simulink library "speedgoatlib_evse"  (R2024b)
settings: Solver=VariableStepAuto  StartTime=0.0  StopTime=10.0  RelTol=1e-3
undefined symbols (not defined in the file): sg_ev_charging_read_m, sg_ev_charging_write_m, sg_ev_isolation_read_m, sg_ev_parameter_read_m, sg_ev_parameter_write_m, sg_ev_precharge_read_m, sg_ev_precharge_write_m, sg_ev_status_m, sg_ev_stop_read_m, sg_ev_stop_write_m, sg_ev_welding_read_m, sg_ev_welding_write_m, sg_evse_charging_read_m, sg_evse_charging_write_m, sg_evse_isolation_read_m, sg_evse_isolation_write_m, sg_evse_parameter_read_m, sg_evse_parameter_write_m, sg_evse_precharge_read_m, sg_evse_precharge_write_m, sg_evse_status_m, sg_evse_stop_read_m, sg_evse_stop_write_m, sg_evse_welding_read_m, sg_evse_welding_write_m
libraries: speedgoatlib_mqtt x199, simulink x39, $bdroot x24
(part 4 of 8)

== system speedgoatlib_evse/Blocks by Charge State/EV Charging Write /string compare logic ==
  Input : Inport
  ASCII to String1 : ASCIIToString
  Add : Sum
  Gain : Gain  Gain=2
  String Compare : StringCompare
  String Compare1 : StringCompare
  String Constant : StringConstant  String="\"started\""
  String Constant1 : StringConstant  String="\"finished\""
  Out1 : Outport
  wires:
  Input/1 -> ASCII to String1/1
  Add/1 -> Out1/1
  Gain/1 -> Add/2
  String Compare1/1 -> Gain/1
  String Constant/1 -> String Compare/2
  String Compare/1 -> Add/1
  String Constant1/1 -> String Compare1/2
  ASCII to String1/1 -> String Compare/1, String Compare1/1

== system speedgoatlib_evse/Blocks by Charge State/EV Charging Write /string compare logic1 ==
  Input : Inport
  ASCII to String1 : ASCIIToString
  Add : Sum
  Gain : Gain  Gain=2
  String Compare : StringCompare
  String Compare1 : StringCompare
  String Constant : StringConstant  String="\"started\""
  String Constant1 : StringConstant  String="\"finished\""
  Out1 : Outport
  wires:
  Input/1 -> ASCII to String1/1
  Add/1 -> Out1/1
  Gain/1 -> Add/2
  String Compare1/1 -> Gain/1
  String Constant/1 -> String Compare/2
  String Compare/1 -> Add/1
  String Constant1/1 -> String Compare1/2
  ASCII to String1/1 -> String Compare/1, String Compare1/1

== system speedgoatlib_evse/Blocks by Charge State/EV Charging Write /string compare logic2 ==
  Input : Inport
  ASCII to String1 : ASCIIToString
  Add : Sum
  Gain : Gain  Gain=2
  String Compare : StringCompare
  String Compare1 : StringCompare
  String Constant : StringConstant  String="\"started\""
  String Constant1 : StringConstant  String="\"finished\""
  Out1 : Outport
  wires:
  ASCII to String1/1 -> String Compare1/1, String Compare/1
  String Constant1/1 -> String Compare1/2
  String Compare/1 -> Add/1
  String Constant/1 -> String Compare/2
  String Compare1/1 -> Gain/1
  Gain/1 -> Add/2
  Add/1 -> Out1/1
  Input/1 -> ASCII to String1/1

== system speedgoatlib_evse/Blocks by Charge State/EV Isolation Read /Enabled Subsystem ==
  Enable : EnablePort
  ASCII to String : ASCIIToString
  ASCII to String1 : ASCIIToString
  ASCII to String2 : ASCIIToString
  Data Type Conversion3 : DataTypeConversion  OutDataTypeStr=boolean  SaturateOnIntegerOverflow=off  RndMeth=Floor
  Data Type Conversion4 : DataTypeConversion  OutDataTypeStr=boolean  SaturateOnIntegerOverflow=off  RndMeth=Floor
  String to Double : ScanString  Format="\"%lf\""
  String to Double1 : ScanString  Format="\"%lf\""
  String to Double2 : ScanString  Format="\"%lf\""
  port0_ci_evse_isolation_evseprocessing : speedgoatlib_mqtt/Client/MQTT Client Subscribe  ClientId=parClientId  ConnectionId=parConnectionId  Topic='port0/ci/evse/isolation/evseprocessing'  QoS=0 - at most once  InitValue=zeros(1,12,'uint8')  Extended=off  SampleTime=parSampleTime
      settings: SourceProductName=MQTT
  port0_ci_evse_isolation_isolationstatus : speedgoatlib_mqtt/Client/MQTT Client Subscribe  ClientId=parClientId  ConnectionId=parConnectionId  Topic='port0/ci/evse/isolation/isolationstatus'  QoS=0 - at most once  InitValue=zeros(1,12,'uint8')  Extended=off  SampleTime=parSampleTime
      settings: SourceProductName=MQTT
  port0_ci_evse_isolation_statuscode : speedgoatlib_mqtt/Client/MQTT Client Subscribe  ClientId=parClientId  ConnectionId=parConnectionId  Topic='port0/ci/evse/isolation/statuscode'  QoS=0 - at most once  InitValue=zeros(1,12,'uint8')  Extended=off  SampleTime=parSampleTime
      settings: SourceProductName=MQTT
  EVSE Processing : Outport
  EVSE Isolationstatus : Outport  Port=2
  EVSE Statuscode : Outport  Port=3
  wires:
  Data Type Conversion4/1 -> EVSE Isolationstatus/1
  port0_ci_evse_isolation_isolationstatus/1 -> ASCII to String2/1
  port0_ci_evse_isolation_statuscode/1 -> ASCII to String1/1
  Data Type Conversion3/1 -> EVSE Statuscode/1
  String to Double/1 -> Data Type Conversion3/1
  ASCII to String1/1 -> String to Double/1
  ASCII to String2/1 -> String to Double1/1
  String to Double1/1 -> Data Type Conversion4/1
  port0_ci_evse_isolation_evseprocessing/1 -> ASCII to String/1
  String to Double2/1 -> EVSE Processing/1
  ASCII to String/1 -> String to Double2/1

== system speedgoatlib_evse/Blocks by Charge State/EV Isolation Read /string compare logic1 ==
  Input : Inport
  ASCII to String1 : ASCIIToString
  Add : Sum
  Gain : Gain  Gain=2
  String Compare : StringCompare
  String Compare1 : StringCompare
  String Constant : StringConstant  String="\"started\""
  String Constant1 : StringConstant  String="\"finished\""
  Out1 : Outport
  wires:
  ASCII to String1/1 -> String Compare1/1, String Compare/1
  String Constant1/1 -> String Compare1/2
  String Compare/1 -> Add/1
  String Constant/1 -> String Compare/2
  String Compare1/1 -> Gain/1
  Gain/1 -> Add/2
  Add/1 -> Out1/1
  Input/1 -> ASCII to String1/1

== system speedgoatlib_evse/Blocks by Charge State/EV Isolation Write /Enabled Subsystem ==
  ready : Inport
  errorcode : Inport  Port=2
  resssoc : Inport  Port=3
  Enable : EnablePort
  Constant1 : Constant  Value=parEnErrorCode  OutDataTypeStr=boolean
  Constant11 : Constant  Value=parEnReady  OutDataTypeStr=boolean
  Constant2 : Constant  Value=parEnRessSoc  OutDataTypeStr=boolean
  Ground1 : Ground
  Ground11 : Ground
  Ground2 : Ground
  String to ASCII : StringToASCII  OutputVectorSize=12
  String to ASCII1 : StringToASCII  OutputVectorSize=24
  String to ASCII2 : StringToASCII  OutputVectorSize=12
  To String : ToString
  To String1 : ToString
  To String2 : ToString
  port0_ci_ev_isolation_errorcode : speedgoatlib_mqtt/Client/MQTT Client Publish  ClientId=parClientId  ConnectionId=parConnectionId  Topic='port0/ci/ev/isolation/errorcode'  QoS=0 - at most once  Retain=on  Extended=on  SampleTime=parSampleTime
      settings: SourceProductName=MQTT
  port0_ci_ev_isolation_ready : speedgoatlib_mqtt/Client/MQTT Client Publish  ClientId=parClientId  ConnectionId=parConnectionId  Topic='port0/ci/ev/isolation/ready'  QoS=0 - at most once  Retain=on  Extended=on  SampleTime=parSampleTime
      settings: SourceProductName=MQTT
  port0_ci_ev_isolation_resssoc : speedgoatlib_mqtt/Client/MQTT Client Publish  ClientId=parClientId  ConnectionId=parConnectionId  Topic='port0/ci/ev/isolation/resssoc'  QoS=0 - at most once  Retain=on  Extended=on  SampleTime=parSampleTime
      settings: SourceProductName=MQTT
  wires:
  Ground2/1 -> port0_ci_ev_isolation_resssoc/3
  Constant2/1 -> port0_ci_ev_isolation_resssoc/2
  Constant1/1 -> port0_ci_ev_isolation_errorcode/2
  Ground1/1 -> port0_ci_ev_isolation_errorcode/3
  Ground11/1 -> port0_ci_ev_isolation_ready/3
  Constant11/1 -> port0_ci_ev_isolation_ready/2
  String to ASCII/1 -> port0_ci_ev_isolation_ready/1
  To String/1 -> String to ASCII/1
  ready/1 -> To String/1
  To String1/1 -> String to ASCII1/1
  String to ASCII1/1 -> port0_ci_ev_isolation_errorcode/1
  String to ASCII2/1 -> port0_ci_ev_isolation_resssoc/1
  To String2/1 -> String to ASCII2/1
  resssoc/1 -> To String2/1
  errorcode/1 -> To String1/1

== system speedgoatlib_evse/Blocks by Charge State/EV Isolation Write /string compare logic ==
  Input : Inport
  ASCII to String1 : ASCIIToString
  Add : Sum
  Gain : Gain  Gain=2
  String Compare : StringCompare
  String Compare1 : StringCompare
  String Constant : StringConstant  String="\"started\""
  String Constant1 : StringConstant  String="\"finished\""
  Out1 : Outport
  wires:
  ASCII to String1/1 -> String Compare1/1, String Compare/1
  String Constant1/1 -> String Compare1/2
  String Compare/1 -> Add/1
  String Constant/1 -> String Compare/2
  String Compare1/1 -> Gain/1
  Gain/1 -> Add/2
  Add/1 -> Out1/1
  Input/1 -> ASCII to String1/1

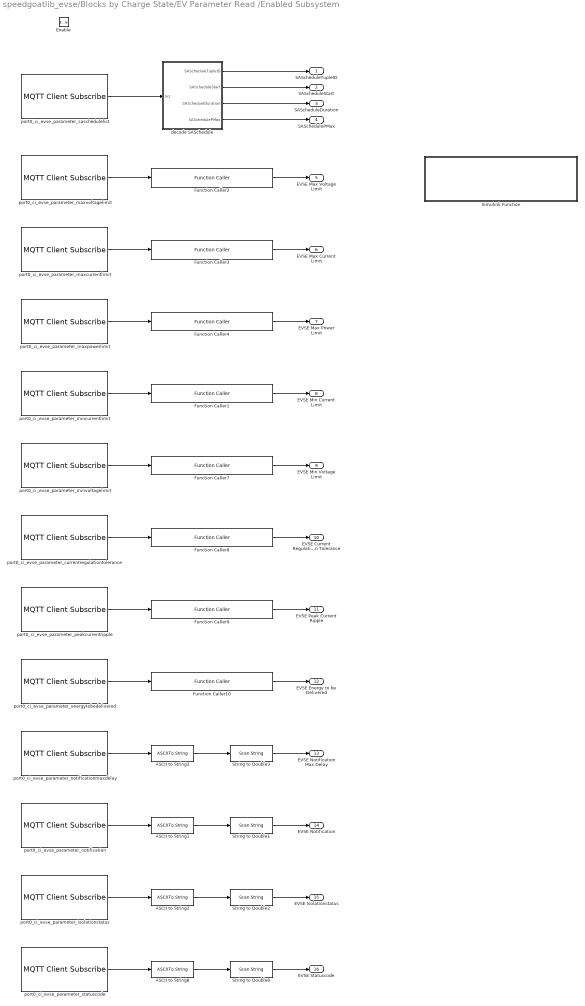
== system speedgoatlib_evse/Blocks by Charge State/EV Parameter Read /Enabled Subsystem ==
  Enable : EnablePort
  ASCII to String{1..3,8} (4 alike) : ASCIIToString
  Function Caller{1..4,7..10} (8 alike) : FunctionCaller  FunctionPrototype=value = fromJsonPhysicalValue(uint8_vec)  InputArgumentSpecifications=zeros(1,48,'uint8')  OutputArgumentSpecifications=double(0)
  Simulink Function : Subsystem  TreatAsAtomicUnit=on
  String to Double{1..3,8} (4 alike) : ScanString  Format="\"%lf\""
  decode SASchedule : Subsystem
  port0_ci_evse_parameter_currentregulationtolerance : speedgoatlib_mqtt/Client/MQTT Client Subscribe  ClientId=parClientId  ConnectionId=parConnectionId  Topic='port0/ci/evse/parameter/currentregulationtolerance'  QoS=0 - at most once  InitValue=zeros(1,48,'uint8')  Extended=off  SampleTime=parSampleTime
      settings: SourceProductName=MQTT
  port0_ci_evse_parameter_energytobedelivered : speedgoatlib_mqtt/Client/MQTT Client Subscribe  ClientId=parClientId  ConnectionId=parConnectionId  Topic='port0/ci/evse/parameter/energytobedelivered'  QoS=0 - at most once  InitValue=zeros(1,48,'uint8')  Extended=off  SampleTime=parSampleTime
      settings: SourceProductName=MQTT
  port0_ci_evse_parameter_isolationstatus : speedgoatlib_mqtt/Client/MQTT Client Subscribe  ClientId=parClientId  ConnectionId=parConnectionId  Topic='port0/ci/evse/parameter/isolationstatus'  QoS=0 - at most once  InitValue=zeros(1,12,'uint8')  Extended=off  SampleTime=parSampleTime
      settings: SourceProductName=MQTT
  port0_ci_evse_parameter_maxcurrentlimit : speedgoatlib_mqtt/Client/MQTT Client Subscribe  ClientId=parClientId  ConnectionId=parConnectionId  Topic='port0/ci/evse/parameter/maxcurrentlimit'  QoS=0 - at most once  InitValue=zeros(1,48,'uint8')  Extended=off  SampleTime=parSampleTime
      settings: SourceProductName=MQTT
  port0_ci_evse_parameter_maxpowerlimit : speedgoatlib_mqtt/Client/MQTT Client Subscribe  ClientId=parClientId  ConnectionId=parConnectionId  Topic='port0/ci/evse/parameter/maxpowerlimit'  QoS=0 - at most once  InitValue=zeros(1,48,'uint8')  Extended=off  SampleTime=parSampleTime
      settings: SourceProductName=MQTT
  port0_ci_evse_parameter_maxvoltagelimit : speedgoatlib_mqtt/Client/MQTT Client Subscribe  ClientId=parClientId  ConnectionId=parConnectionId  Topic='port0/ci/evse/parameter/maxvoltagelimit'  QoS=0 - at most once  InitValue=zeros(1,48,'uint8')  Extended=off  SampleTime=parSampleTime
      settings: SourceProductName=MQTT
  port0_ci_evse_parameter_mincurrentlimit : speedgoatlib_mqtt/Client/MQTT Client Subscribe  ClientId=parClientId  ConnectionId=parConnectionId  Topic='port0/ci/evse/parameter/mincurrentlimit'  QoS=0 - at most once  InitValue=zeros(1,48,'uint8')  Extended=off  SampleTime=parSampleTime
      settings: SourceProductName=MQTT
  port0_ci_evse_parameter_minvoltagelimit : speedgoatlib_mqtt/Client/MQTT Client Subscribe  ClientId=parClientId  ConnectionId=parConnectionId  Topic='port0/ci/evse/parameter/minvoltagelimit'  QoS=0 - at most once  InitValue=zeros(1,48,'uint8')  Extended=off  SampleTime=parSampleTime
      settings: SourceProductName=MQTT
  port0_ci_evse_parameter_notification : speedgoatlib_mqtt/Client/MQTT Client Subscribe  ClientId=parClientId  ConnectionId=parConnectionId  Topic='port0/ci/evse/parameter/notification'  QoS=0 - at most once  InitValue=zeros(1,16,'uint8')  Extended=off  SampleTime=parSampleTime
      settings: SourceProductName=MQTT
  port0_ci_evse_parameter_notificationmaxdelay : speedgoatlib_mqtt/Client/MQTT Client Subscribe  ClientId=parClientId  ConnectionId=parConnectionId  Topic='port0/ci/evse/parameter/notificationmaxdelay'  QoS=0 - at most once  InitValue=zeros(1,16,'uint8')  Extended=off  SampleTime=parSampleTime
      settings: SourceProductName=MQTT
  port0_ci_evse_parameter_peakcurrentripple : speedgoatlib_mqtt/Client/MQTT Client Subscribe  ClientId=parClientId  ConnectionId=parConnectionId  Topic='port0/ci/evse/parameter/peakcurrentripple'  QoS=0 - at most once  InitValue=zeros(1,48,'uint8')  Extended=off  SampleTime=parSampleTime
      settings: SourceProductName=MQTT
  port0_ci_evse_parameter_saschedulelist : speedgoatlib_mqtt/Client/MQTT Client Subscribe  ClientId=parClientId  ConnectionId=parConnectionId  Topic='port0/ci/evse/parameter/saschedulelist'  QoS=0 - at most once  InitValue=zeros(1,255,'uint8')  Extended=off  SampleTime=parSampleTime
      settings: SourceProductName=MQTT
  port0_ci_evse_parameter_statuscode : speedgoatlib_mqtt/Client/MQTT Client Subscribe  ClientId=parClientId  ConnectionId=parConnectionId  Topic='port0/ci/evse/parameter/statuscode'  QoS=0 - at most once  InitValue=zeros(1,12,'uint8')  Extended=off  SampleTime=parSampleTime
      settings: SourceProductName=MQTT
  SAScheduleTupleID : Outport
  SAScheduleStart : Outport  Port=2
  SAScheduleDuration : Outport  Port=3
  SASchedulePMax : Outport  Port=4
  EVSE Max Voltage Limit : Outport  Port=5
  EVSE Max Current Limit : Outport  Port=6
  EVSE Max Power Limit : Outport  Port=7
  EVSE Min Current Limit : Outport  Port=8
  EVSE Min Voltage Limit : Outport  Port=9
  EVSE Current Regulation Tolerance : Outport  Port=10
  EVSE Peak Current Ripple : Outport  Port=11
  EVSE Energy to be Delivered : Outport  Port=12
  EVSE Notification Max Delay : Outport  Port=13
  EVSE Notification : Outport  Port=14
  EVSE Isolationstatus : Outport  Port=15
  EVSE Statuscode : Outport  Port=16
  wires:
  String to Double3/1 -> EVSE Notification Max Delay/1
  ASCII to String3/1 -> String to Double3/1
  port0_ci_evse_parameter_notificationmaxdelay/1 -> ASCII to String3/1
  Function Caller1/1 -> EVSE Min Current Limit/1
  port0_ci_evse_parameter_mincurrentlimit/1 -> Function Caller1/1
  Function Caller2/1 -> EVSE Max Voltage Limit/1
  port0_ci_evse_parameter_maxvoltagelimit/1 -> Function Caller2/1
  port0_ci_evse_parameter_maxcurrentlimit/1 -> Function Caller3/1
  Function Caller3/1 -> EVSE Max Current Limit/1
  Function Caller4/1 -> EVSE Max Power Limit/1
  port0_ci_evse_parameter_maxpowerlimit/1 -> Function Caller4/1
  port0_ci_evse_parameter_saschedulelist/1 -> decode SASchedule/1(In1)
  decode SASchedule/1(SAScheduleTupleID) -> SAScheduleTupleID/1
  decode SASchedule/2(SAScheduleStart) -> SAScheduleStart/1
  decode SASchedule/4(SASchedulePMax) -> SASchedulePMax/1
  decode SASchedule/3(SAScheduelDuration) -> SAScheduleDuration/1
  port0_ci_evse_parameter_minvoltagelimit/1 -> Function Caller7/1
  Function Caller7/1 -> EVSE Min Voltage Limit/1
  port0_ci_evse_parameter_currentregulationtolerance/1 -> Function Caller8/1
  Function Caller8/1 -> EVSE Current Regulation Tolerance/1
  port0_ci_evse_parameter_peakcurrentripple/1 -> Function Caller9/1
  Function Caller9/1 -> EVSE Peak Current Ripple/1
  port0_ci_evse_parameter_energytobedelivered/1 -> Function Caller10/1
  Function Caller10/1 -> EVSE Energy to be Delivered/1
  port0_ci_evse_parameter_notification/1 -> ASCII to String1/1
  ASCII to String1/1 -> String to Double1/1
  String to Double1/1 -> EVSE Notification/1
  String to Double2/1 -> EVSE Isolationstatus/1
  ASCII to String2/1 -> String to Double2/1
  port0_ci_evse_parameter_isolationstatus/1 -> ASCII to String2/1
  port0_ci_evse_parameter_statuscode/1 -> ASCII to String8/1
  ASCII to String8/1 -> String to Double8/1
  String to Double8/1 -> EVSE Statuscode/1

== system speedgoatlib_evse/Blocks by Charge State/EV Parameter Read /string compare logic ==
  Input : Inport
  ASCII to String1 : ASCIIToString
  Add : Sum
  Data Type Conversion : DataTypeConversion  OutDataTypeStr=double  SaturateOnIntegerOverflow=off  RndMeth=Floor
  Data Type Conversion1 : DataTypeConversion  OutDataTypeStr=double  SaturateOnIntegerOverflow=off  RndMeth=Floor
  Gain : Gain  Gain=2
  String Compare : StringCompare
  String Compare1 : StringCompare
  String Constant : StringConstant  String="\"started\""
  String Constant1 : StringConstant  String="\"finished\""
  Out1 : Outport
  wires:
  Input/1 -> ASCII to String1/1
  Add/1 -> Out1/1
  Gain/1 -> Add/2
  String Compare1/1 -> Data Type Conversion1/1
  String Constant/1 -> String Compare/2
  String Compare/1 -> Data Type Conversion/1
  String Constant1/1 -> String Compare1/2
  ASCII to String1/1 -> String Compare/1, String Compare1/1
  Data Type Conversion/1 -> Add/1
  Data Type Conversion1/1 -> Gain/1

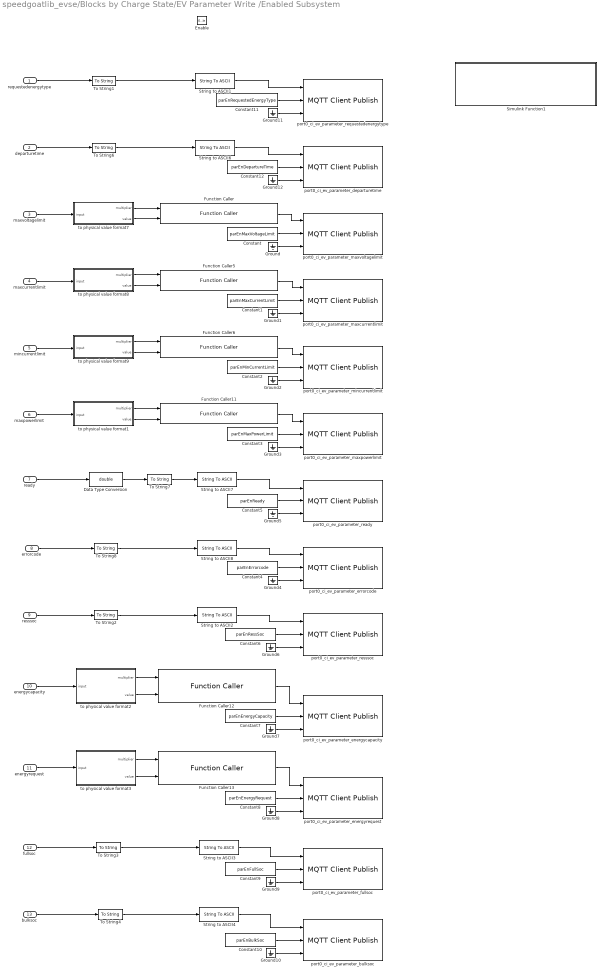
== system speedgoatlib_evse/Blocks by Charge State/EV Parameter Write /Enabled Subsystem ==
  requestedenergytype : Inport
  departuretime : Inport  Port=2
  maxvoltagelimit : Inport  Port=3
  maxcurrentlimit : Inport  Port=4
  mincurrentlimit : Inport  Port=5
  maxpowerlimit : Inport  Port=6
  ready : Inport  Port=7
  errorcode : Inport  Port=8
  resssoc : Inport  Port=9
  energycapacity : Inport  Port=10
  energyrequest : Inport  Port=11
  fullsoc : Inport  Port=12
  bulksoc : Inport  Port=13
  Enable : EnablePort
  Constant : Constant  Value=parEnMaxVoltageLimit  OutDataTypeStr=boolean
  Constant1 : Constant  Value=parEnMaxCurrentLimit  OutDataTypeStr=boolean
  Constant10 : Constant  Value=parEnBulkSoc  OutDataTypeStr=boolean
  Constant11 : Constant  Value=parEnRequestedEnergyType  OutDataTypeStr=boolean
  Constant12 : Constant  Value=parEnDepartureTime  OutDataTypeStr=boolean
  Constant2 : Constant  Value=parEnMinCurrentLimit  OutDataTypeStr=boolean
  Constant3 : Constant  Value=parEnMaxPowerLimit  OutDataTypeStr=boolean
  Constant4 : Constant  Value=parEnErrorcode  OutDataTypeStr=boolean
  Constant5 : Constant  Value=parEnReady  OutDataTypeStr=boolean
  Constant6 : Constant  Value=parEnRessSoc  OutDataTypeStr=boolean
  Constant7 : Constant  Value=parEnEnergyCapacity  OutDataTypeStr=boolean
  Constant8 : Constant  Value=parEnEnergyRequest  OutDataTypeStr=boolean
  Constant9 : Constant  Value=parEnFullSoc  OutDataTypeStr=boolean
  Data Type Conversion : DataTypeConversion  OutDataTypeStr=double  SaturateOnIntegerOverflow=off  RndMeth=Floor
  Function Caller{,5..6,11..13} (6 alike) : FunctionCaller  FunctionPrototype=json_string = toJsonPhysicalValue(multiplier,value)  InputArgumentSpecifications=double(0), double(0)  OutputArgumentSpecifications=zeros(1,48,'uint8')
  Ground{,1..12} (13 alike) : Ground
  Simulink Function1 : Subsystem  TreatAsAtomicUnit=on
  String to ASCII{1..4,7} (5 alike) : StringToASCII  OutputVectorSize=12
  String to ASCII6 : StringToASCII  OutputVectorSize=24
  String to ASCII8 : StringToASCII  OutputVectorSize=24
  To String{1..4,6..8} (7 alike) : ToString
  port0_ci_ev_parameter_bulksoc : speedgoatlib_mqtt/Client/MQTT Client Publish  ClientId=parClientId  ConnectionId=parConnectionId  Topic='port0/ci/ev/parameter/bulksoc'  QoS=0 - at most once  Retain=on  Extended=on  SampleTime=parSampleTime
      settings: SourceProductName=MQTT
  port0_ci_ev_parameter_departuretime : speedgoatlib_mqtt/Client/MQTT Client Publish  ClientId=parClientId  ConnectionId=parConnectionId  Topic='port0/ci/ev/parameter/departuretime'  QoS=0 - at most once  Retain=on  Extended=on  SampleTime=parSampleTime
      settings: SourceProductName=MQTT
  port0_ci_ev_parameter_energycapacity : speedgoatlib_mqtt/Client/MQTT Client Publish  ClientId=parClientId  ConnectionId=parConnectionId  Topic='port0/ci/ev/parameter/energycapacity'  QoS=0 - at most once  Retain=on  Extended=on  SampleTime=parSampleTime
      settings: SourceProductName=MQTT
  port0_ci_ev_parameter_energyrequest : speedgoatlib_mqtt/Client/MQTT Client Publish  ClientId=parClientId  ConnectionId=parConnectionId  Topic='port0/ci/ev/parameter/energyrequest'  QoS=0 - at most once  Retain=on  Extended=on  SampleTime=parSampleTime
      settings: SourceProductName=MQTT
  port0_ci_ev_parameter_errorcode : speedgoatlib_mqtt/Client/MQTT Client Publish  ClientId=parClientId  ConnectionId=parConnectionId  Topic='port0/ci/ev/parameter/errorcode'  QoS=0 - at most once  Retain=on  Extended=on  SampleTime=parSampleTime
      settings: SourceProductName=MQTT
  port0_ci_ev_parameter_fullsoc : speedgoatlib_mqtt/Client/MQTT Client Publish  ClientId=parClientId  ConnectionId=parConnectionId  Topic='port0/ci/ev/parameter/fullsoc'  QoS=0 - at most once  Retain=on  Extended=on  SampleTime=parSampleTime
      settings: SourceProductName=MQTT
  port0_ci_ev_parameter_maxcurrentlimit : speedgoatlib_mqtt/Client/MQTT Client Publish  ClientId=parClientId  ConnectionId=parConnectionId  Topic='port0/ci/ev/parameter/maxcurrentlimit'  QoS=0 - at most once  Retain=on  Extended=on  SampleTime=parSampleTime
      settings: SourceProductName=MQTT
  port0_ci_ev_parameter_maxpowerlimit : speedgoatlib_mqtt/Client/MQTT Client Publish  ClientId=parClientId  ConnectionId=parConnectionId  Topic='port0/ci/ev/parameter/maxpowerlimit'  QoS=0 - at most once  Retain=on  Extended=on  SampleTime=parSampleTime
      settings: SourceProductName=MQTT
  port0_ci_ev_parameter_maxvoltagelimit : speedgoatlib_mqtt/Client/MQTT Client Publish  ClientId=parClientId  ConnectionId=parConnectionId  Topic='port0/ci/ev/parameter/maxvoltagelimit'  QoS=0 - at most once  Retain=on  Extended=on  SampleTime=parSampleTime
      settings: SourceProductName=MQTT
  port0_ci_ev_parameter_mincurrentlimit : speedgoatlib_mqtt/Client/MQTT Client Publish  ClientId=parClientId  ConnectionId=parConnectionId  Topic='port0/ci/ev/parameter/mincurrentlimit'  QoS=0 - at most once  Retain=on  Extended=on  SampleTime=parSampleTime
      settings: SourceProductName=MQTT
  port0_ci_ev_parameter_ready : speedgoatlib_mqtt/Client/MQTT Client Publish  ClientId=parClientId  ConnectionId=parConnectionId  Topic='port0/ci/ev/parameter/ready'  QoS=0 - at most once  Retain=on  Extended=on  SampleTime=parSampleTime
      settings: SourceProductName=MQTT
  port0_ci_ev_parameter_requestedenergytype : speedgoatlib_mqtt/Client/MQTT Client Publish  ClientId=parClientId  ConnectionId=parConnectionId  Topic='port0/ci/ev/parameter/requestedenergytype'  QoS=0 - at most once  Retain=on  Extended=on  SampleTime=parSampleTime
      settings: SourceProductName=MQTT
  port0_ci_ev_parameter_resssoc : speedgoatlib_mqtt/Client/MQTT Client Publish  ClientId=parClientId  ConnectionId=parConnectionId  Topic='port0/ci/ev/parameter/resssoc'  QoS=0 - at most once  Retain=on  Extended=on  SampleTime=parSampleTime
      settings: SourceProductName=MQTT
  to physical value format1 : MATLAB Function  TreatAsAtomicUnit=on
  to physical value format2 : MATLAB Function  TreatAsAtomicUnit=on
  to physical value format3 : MATLAB Function  TreatAsAtomicUnit=on
  to physical value format7 : MATLAB Function  TreatAsAtomicUnit=on
  to physical value format8 : MATLAB Function  TreatAsAtomicUnit=on
  to physical value format9 : MATLAB Function  TreatAsAtomicUnit=on
  wires:
  to physical value format3/1(multiplier) -> Function Caller13/1
  to physical value format3/2(value) -> Function Caller13/2
  Function Caller13/1 -> port0_ci_ev_parameter_energyrequest/1
  Function Caller12/1 -> port0_ci_ev_parameter_energycapacity/1
  to physical value format2/2(value) -> Function Caller12/2
  to physical value format2/1(multiplier) -> Function Caller12/1
  Ground4/1 -> port0_ci_ev_parameter_errorcode/3
  Constant4/1 -> port0_ci_ev_parameter_errorcode/2
  Constant3/1 -> port0_ci_ev_parameter_maxpowerlimit/2
  Ground3/1 -> port0_ci_ev_parameter_maxpowerlimit/3
  Function Caller11/1 -> port0_ci_ev_parameter_maxpowerlimit/1
  to physical value format1/1(multiplier) -> Function Caller11/1
  to physical value format1/2(value) -> Function Caller11/2
  to physical value format9/2(value) -> Function Caller6/2
  to physical value format9/1(multiplier) -> Function Caller6/1
  Function Caller6/1 -> port0_ci_ev_parameter_mincurrentlimit/1
  Ground2/1 -> port0_ci_ev_parameter_mincurrentlimit/3
  Constant2/1 -> port0_ci_ev_parameter_mincurrentlimit/2
  Constant1/1 -> port0_ci_ev_parameter_maxcurrentlimit/2
  Ground1/1 -> port0_ci_ev_parameter_maxcurrentlimit/3
  Function Caller5/1 -> port0_ci_ev_parameter_maxcurrentlimit/1
  to physical value format8/1(multiplier) -> Function Caller5/1
  to physical value format8/2(value) -> Function Caller5/2
  to physical value format7/2(value) -> Function Caller/2
  to physical value format7/1(multiplier) -> Function Caller/1
  Function Caller/1 -> port0_ci_ev_parameter_maxvoltagelimit/1
  Ground/1 -> port0_ci_ev_parameter_maxvoltagelimit/3
  Constant/1 -> port0_ci_ev_parameter_maxvoltagelimit/2
  String to ASCII4/1 -> port0_ci_ev_parameter_bulksoc/1
  To String4/1 -> String to ASCII4/1
  bulksoc/1 -> To String4/1
  fullsoc/1 -> To String3/1
  To String3/1 -> String to ASCII3/1
  String to ASCII3/1 -> port0_ci_ev_parameter_fullsoc/1
  energyrequest/1 -> to physical value format3/1(input)
  energycapacity/1 -> to physical value format2/1(input)
  String to ASCII2/1 -> port0_ci_ev_parameter_resssoc/1
  To String2/1 -> String to ASCII2/1
  resssoc/1 -> To String2/1
  errorcode/1 -> To String8/1
  To String8/1 -> String to ASCII8/1
  String to ASCII8/1 -> port0_ci_ev_parameter_errorcode/1
  Data Type Conversion/1 -> To String7/1
  ready/1 -> Data Type Conversion/1
  To String7/1 -> String to ASCII7/1
  String to ASCII7/1 -> port0_ci_ev_parameter_ready/1
  String to ASCII6/1 -> port0_ci_ev_parameter_departuretime/1
  To String6/1 -> String to ASCII6/1
  departuretime/1 -> To String6/1
  To String1/1 -> String to ASCII1/1
  requestedenergytype/1 -> To String1/1
  String to ASCII1/1 -> port0_ci_ev_parameter_requestedenergytype/1
  maxvoltagelimit/1 -> to physical value format7/1(input)
  maxcurrentlimit/1 -> to physical value format8/1(input)
  mincurrentlimit/1 -> to physical value format9/1(input)
  maxpowerlimit/1 -> to physical value format1/1(input)
  Ground5/1 -> port0_ci_ev_parameter_ready/3
  Constant5/1 -> port0_ci_ev_parameter_ready/2
  Constant6/1 -> port0_ci_ev_parameter_resssoc/2
  Ground6/1 -> port0_ci_ev_parameter_resssoc/3
  Ground7/1 -> port0_ci_ev_parameter_energycapacity/3
  Constant7/1 -> port0_ci_ev_parameter_energycapacity/2
  Constant8/1 -> port0_ci_ev_parameter_energyrequest/2
  Ground8/1 -> port0_ci_ev_parameter_energyrequest/3
  Ground9/1 -> port0_ci_ev_parameter_fullsoc/3
  Constant9/1 -> port0_ci_ev_parameter_fullsoc/2
  Constant10/1 -> port0_ci_ev_parameter_bulksoc/2
  Ground10/1 -> port0_ci_ev_parameter_bulksoc/3
  Constant11/1 -> port0_ci_ev_parameter_requestedenergytype/2
  Ground11/1 -> port0_ci_ev_parameter_requestedenergytype/3
  Constant12/1 -> port0_ci_ev_parameter_departuretime/2
  Ground12/1 -> port0_ci_ev_parameter_departuretime/3

== system speedgoatlib_evse/Blocks by Charge State/EV Parameter Write /string compare logic ==
  Input : Inport
  ASCII to String1 : ASCIIToString
  Add : Sum
  Data Type Conversion : DataTypeConversion  OutDataTypeStr=double  SaturateOnIntegerOverflow=off  RndMeth=Floor
  Data Type Conversion1 : DataTypeConversion  OutDataTypeStr=double  SaturateOnIntegerOverflow=off  RndMeth=Floor
  Gain : Gain  Gain=2
  String Compare : StringCompare
  String Compare1 : StringCompare
  String Constant : StringConstant  String="\"started\""
  String Constant1 : StringConstant  String="\"finished\""
  Out1 : Outport
  wires:
  ASCII to String1/1 -> String Compare1/1, String Compare/1
  String Constant1/1 -> String Compare1/2
  String Compare/1 -> Data Type Conversion/1
  String Constant/1 -> String Compare/2
  String Compare1/1 -> Data Type Conversion1/1
  Gain/1 -> Add/2
  Add/1 -> Out1/1
  Input/1 -> ASCII to String1/1
  Data Type Conversion/1 -> Add/1
  Data Type Conversion1/1 -> Gain/1

== system speedgoatlib_evse/Blocks by Charge State/EV Pre-Charge Read /Enabled Subsystem ==
  Enable : EnablePort
  ASCII to String1 : ASCIIToString
  ASCII to String2 : ASCIIToString
  Data Type Conversion3 : DataTypeConversion  OutDataTypeStr=boolean  SaturateOnIntegerOverflow=off  RndMeth=Floor
  Data Type Conversion4 : DataTypeConversion  OutDataTypeStr=boolean  SaturateOnIntegerOverflow=off  RndMeth=Floor
  Function Caller : FunctionCaller  FunctionPrototype=value = fromJsonPhysicalValue(uint8_vec)  InputArgumentSpecifications=zeros(1,48,'uint8')  OutputArgumentSpecifications=double(0)
  Simulink Function : Subsystem  TreatAsAtomicUnit=on
  String to Double : ScanString  Format="\"%lf\""
  String to Double1 : ScanString  Format="\"%lf\""
  port0_ci_evse_charge_presentvoltage : speedgoatlib_mqtt/Client/MQTT Client Subscribe  ClientId=parClientId  ConnectionId=parConnectionId  Topic='port0/ci/evse/charge/presentvoltage'  QoS=0 - at most once  InitValue=zeros(1,48,'uint8')  Extended=off  SampleTime=parSampleTime
      settings: SourceProductName=MQTT
  port0_ci_evse_parameter_isolationstatus : speedgoatlib_mqtt/Client/MQTT Client Subscribe  ClientId=parClientId  ConnectionId=parConnectionId  Topic='port0/ci/evse/parameter/isolationstatus'  QoS=0 - at most once  InitValue=zeros(1,12,'uint8')  Extended=off  SampleTime=parSampleTime
      settings: SourceProductName=MQTT
  port0_ci_evse_parameter_statuscode : speedgoatlib_mqtt/Client/MQTT Client Subscribe  ClientId=parClientId  ConnectionId=parConnectionId  Topic='port0/ci/evse/parameter/statuscode'  QoS=0 - at most once  InitValue=zeros(1,12,'uint8')  Extended=off  SampleTime=parSampleTime
      settings: SourceProductName=MQTT
  EVSE Isolationstatus : Outport
  EVSE Statuscode : Outport  Port=2
  EVSE Present Voltage : Outport  Port=3
  wires:
  Data Type Conversion4/1 -> EVSE Isolationstatus/1
  port0_ci_evse_parameter_isolationstatus/1 -> ASCII to String2/1
  port0_ci_evse_parameter_statuscode/1 -> ASCII to String1/1
  Data Type Conversion3/1 -> EVSE Statuscode/1
  port0_ci_evse_charge_presentvoltage/1 -> Function Caller/1
  Function Caller/1 -> EVSE Present Voltage/1
  String to Double/1 -> Data Type Conversion3/1
  ASCII to String1/1 -> String to Double/1
  ASCII to String2/1 -> String to Double1/1
  String to Double1/1 -> Data Type Conversion4/1

== system speedgoatlib_evse/Blocks by Charge State/EV Pre-Charge Read /string compare logic1 ==
  Input : Inport
  ASCII to String1 : ASCIIToString
  Add : Sum
  Gain : Gain  Gain=2
  String Compare : StringCompare
  String Compare1 : StringCompare
  String Constant : StringConstant  String="\"started\""
  String Constant1 : StringConstant  String="\"finished\""
  Out1 : Outport
  wires:
  ASCII to String1/1 -> String Compare1/1, String Compare/1
  String Constant1/1 -> String Compare1/2
  String Compare/1 -> Add/1
  String Constant/1 -> String Compare/2
  String Compare1/1 -> Gain/1
  Gain/1 -> Add/2
  Add/1 -> Out1/1
  Input/1 -> ASCII to String1/1

== system speedgoatlib_evse/Blocks by Charge State/EV Pre-Charge Write /Enabled Subsystem ==
  ready : Inport
  errorcode : Inport  Port=2
  resssoc : Inport  Port=3
  targetvoltage : Inport  Port=4
  targetcurrent : Inport  Port=5
  Enable : EnablePort
  Constant1 : Constant  Value=parEnErrorCode  OutDataTypeStr=boolean
  Constant11 : Constant  Value=parEnReady  OutDataTypeStr=boolean
  Constant2 : Constant  Value=parEnRessSoc  OutDataTypeStr=boolean
  Constant3 : Constant  Value=parEnTargetVoltage  OutDataTypeStr=boolean
  Constant4 : Constant  Value=parEnTargetCurrent  OutDataTypeStr=boolean
  Function Caller13 : FunctionCaller  FunctionPrototype=json_string = toJsonPhysicalValue(multiplier,value)  InputArgumentSpecifications=double(0), double(0)  OutputArgumentSpecifications=zeros(1,48,'uint8')
  Function Caller5 : FunctionCaller  FunctionPrototype=json_string = toJsonPhysicalValue(multiplier,value)  InputArgumentSpecifications=double(0), double(0)  OutputArgumentSpecifications=zeros(1,48,'uint8')
  Ground{1..4,11} (5 alike) : Ground
  Simulink Function1 : Subsystem  TreatAsAtomicUnit=on
  String to ASCII : StringToASCII  OutputVectorSize=12
  String to ASCII1 : StringToASCII  OutputVectorSize=24
  String to ASCII2 : StringToASCII  OutputVectorSize=12
  To String : ToString
  To String1 : ToString
  To String2 : ToString
  port0_ci_ev_precharge_errorcode : speedgoatlib_mqtt/Client/MQTT Client Publish  ClientId=parClientId  ConnectionId=parConnectionId  Topic='port0/ci/ev/precharge/errorcode'  QoS=0 - at most once  Retain=on  Extended=on  SampleTime=parSampleTime
      settings: SourceProductName=MQTT
  port0_ci_ev_precharge_ready : speedgoatlib_mqtt/Client/MQTT Client Publish  ClientId=parClientId  ConnectionId=parConnectionId  Topic='port0/ci/ev/precharge/ready'  QoS=0 - at most once  Retain=on  Extended=on  SampleTime=parSampleTime
      settings: SourceProductName=MQTT
  port0_ci_ev_precharge_resssoc : speedgoatlib_mqtt/Client/MQTT Client Publish  ClientId=parClientId  ConnectionId=parConnectionId  Topic='port0/ci/ev/precharge/resssoc'  QoS=0 - at most once  Retain=on  Extended=on  SampleTime=parSampleTime
      settings: SourceProductName=MQTT
  port0_ci_ev_precharge_targetcurrent : speedgoatlib_mqtt/Client/MQTT Client Publish  ClientId=parClientId  ConnectionId=parConnectionId  Topic='port0/ci/ev/precharge/targetcurrent'  QoS=0 - at most once  Retain=on  Extended=on  SampleTime=parSampleTime
      settings: SourceProductName=MQTT
  port0_ci_ev_precharge_targetvoltage : speedgoatlib_mqtt/Client/MQTT Client Publish  ClientId=parClientId  ConnectionId=parConnectionId  Topic='port0/ci/ev/precharge/targetvoltage'  QoS=0 - at most once  Retain=on  Extended=on  SampleTime=parSampleTime
      settings: SourceProductName=MQTT
  to physical value format : MATLAB Function  TreatAsAtomicUnit=on
  to physical value format1 : MATLAB Function  TreatAsAtomicUnit=on
  wires:
  to physical value format1/1(multiplier) -> Function Caller5/1
  to physical value format1/2(value) -> Function Caller5/2
  Function Caller5/1 -> port0_ci_ev_precharge_targetcurrent/1
  Function Caller13/1 -> port0_ci_ev_precharge_targetvoltage/1
  to physical value format/2(value) -> Function Caller13/2
  to physical value format/1(multiplier) -> Function Caller13/1
  errorcode/1 -> To String1/1
  resssoc/1 -> To String2/1
  To String2/1 -> String to ASCII2/1
  String to ASCII2/1 -> port0_ci_ev_precharge_resssoc/1
  String to ASCII1/1 -> port0_ci_ev_precharge_errorcode/1
  To String1/1 -> String to ASCII1/1
  ready/1 -> To String/1
  To String/1 -> String to ASCII/1
  String to ASCII/1 -> port0_ci_ev_precharge_ready/1
  targetcurrent/1 -> to physical value format1/1(input)
  targetvoltage/1 -> to physical value format/1(input)
  Constant11/1 -> port0_ci_ev_precharge_ready/2
  Ground11/1 -> port0_ci_ev_precharge_ready/3
  Ground1/1 -> port0_ci_ev_precharge_errorcode/3
  Constant1/1 -> port0_ci_ev_precharge_errorcode/2
  Constant2/1 -> port0_ci_ev_precharge_resssoc/2
  Ground2/1 -> port0_ci_ev_precharge_resssoc/3
  Ground3/1 -> port0_ci_ev_precharge_targetvoltage/3
  Constant3/1 -> port0_ci_ev_precharge_targetvoltage/2
  Constant4/1 -> port0_ci_ev_precharge_targetcurrent/2
  Ground4/1 -> port0_ci_ev_precharge_targetcurrent/3

== system speedgoatlib_evse/Blocks by Charge State/EV Pre-Charge Write /string compare logic ==
  Input : Inport
  ASCII to String1 : ASCIIToString
  Add : Sum
  Gain : Gain  Gain=2
  String Compare : StringCompare
  String Compare1 : StringCompare
  String Constant : StringConstant  String="\"started\""
  String Constant1 : StringConstant  String="\"finished\""
  Out1 : Outport
  wires:
  Input/1 -> ASCII to String1/1
  Add/1 -> Out1/1
  Gain/1 -> Add/2
  String Compare1/1 -> Gain/1
  String Constant/1 -> String Compare/2
  String Compare/1 -> Add/1
  String Constant1/1 -> String Compare1/2
  ASCII to String1/1 -> String Compare/1, String Compare1/1

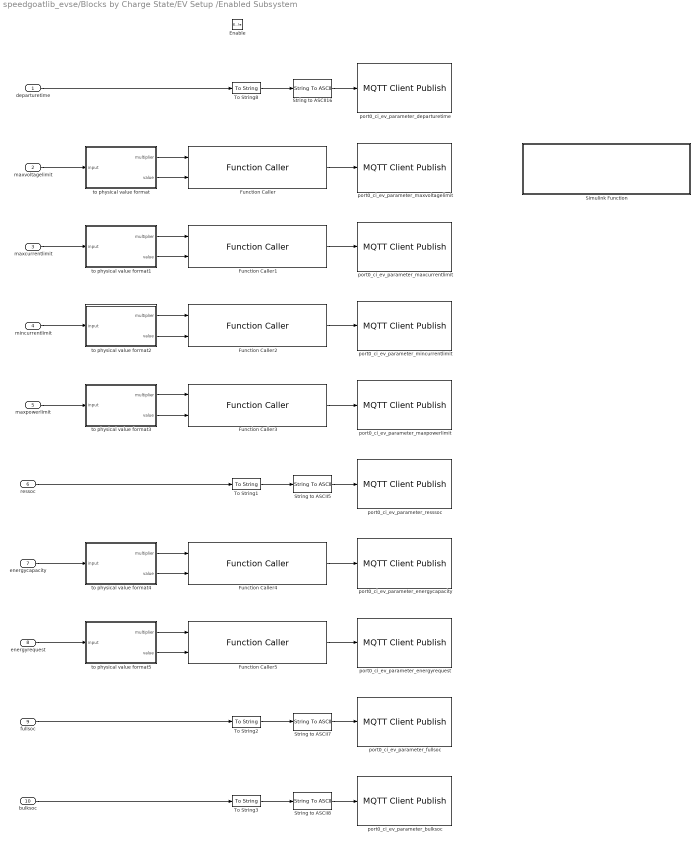
== system speedgoatlib_evse/Blocks by Charge State/EV Setup /Enabled Subsystem ==
  departuretime : Inport
  maxvoltagelimit : Inport  Port=2
  maxcurrentlimit : Inport  Port=3
  mincurrentlimit : Inport  Port=4
  maxpowerlimit : Inport  Port=5
  ressoc : Inport  Port=6
  energycapacity : Inport  Port=7
  energyrequest : Inport  Port=8
  fullsoc : Inport  Port=9
  bulksoc : Inport  Port=10
  Enable : EnablePort
  Function Caller{,1..5} (6 alike) : FunctionCaller  FunctionPrototype=json_string = toJsonPhysicalValue(multiplier,value)  InputArgumentSpecifications=double(0), double(0)  OutputArgumentSpecifications=zeros(1,48,'uint8')
  Simulink Function : Subsystem  TreatAsAtomicUnit=on
  String to ASCII16 : StringToASCII
  String to ASCII5 : StringToASCII  OutputVectorSize=12
  String to ASCII7 : StringToASCII  OutputVectorSize=12
  String to ASCII8 : StringToASCII  OutputVectorSize=12
  To String{1..3,8} (4 alike) : ToString
  port0_ci_ev_parameter_bulksoc : speedgoatlib_mqtt/Client/MQTT Client Publish  ClientId=parClientId  ConnectionId=parConnectionId  Topic='port0/ci/ev/parameter/bulksoc'  QoS=0 - at most once  Retain=on  Extended=off  SampleTime=parSampleTime
      settings: SourceProductName=MQTT
  port0_ci_ev_parameter_departuretime : speedgoatlib_mqtt/Client/MQTT Client Publish  ClientId=parClientId  ConnectionId=parConnectionId  Topic='port0/ci/ev/parameter/departuretime'  QoS=0 - at most once  Retain=on  Extended=off  SampleTime=parSampleTime
      settings: SourceProductName=MQTT
  port0_ci_ev_parameter_energycapacity : speedgoatlib_mqtt/Client/MQTT Client Publish  ClientId=parClientId  ConnectionId=parConnectionId  Topic='port0/ci/ev/parameter/energycapacity'  QoS=0 - at most once  Retain=on  Extended=off  SampleTime=parSampleTime
      settings: SourceProductName=MQTT
  port0_ci_ev_parameter_energyrequest : speedgoatlib_mqtt/Client/MQTT Client Publish  ClientId=parClientId  ConnectionId=parConnectionId  Topic='port0/ci/ev/parameter/energyrequest'  QoS=0 - at most once  Retain=on  Extended=off  SampleTime=parSampleTime
      settings: SourceProductName=MQTT
  port0_ci_ev_parameter_fullsoc : speedgoatlib_mqtt/Client/MQTT Client Publish  ClientId=parClientId  ConnectionId=parConnectionId  Topic='port0/ci/ev/parameter/fullsoc'  QoS=0 - at most once  Retain=on  Extended=off  SampleTime=parSampleTime
      settings: SourceProductName=MQTT
  port0_ci_ev_parameter_maxcurrentlimit : speedgoatlib_mqtt/Client/MQTT Client Publish  ClientId=parClientId  ConnectionId=parConnectionId  Topic='port0/ci/ev/parameter/maxcurrentlimit'  QoS=0 - at most once  Retain=on  Extended=off  SampleTime=parSampleTime
      settings: SourceProductName=MQTT
  port0_ci_ev_parameter_maxpowerlimit : speedgoatlib_mqtt/Client/MQTT Client Publish  ClientId=parClientId  ConnectionId=parConnectionId  Topic='port0/ci/ev/parameter/maxpowerlimit'  QoS=0 - at most once  Retain=on  Extended=off  SampleTime=parSampleTime
      settings: SourceProductName=MQTT
  port0_ci_ev_parameter_maxvoltagelimit : speedgoatlib_mqtt/Client/MQTT Client Publish  ClientId=parClientId  ConnectionId=parConnectionId  Topic='port0/ci/ev/parameter/maxvoltagelimit'  QoS=0 - at most once  Retain=on  Extended=off  SampleTime=parSampleTime
      settings: SourceProductName=MQTT
  port0_ci_ev_parameter_mincurrentlimit : speedgoatlib_mqtt/Client/MQTT Client Publish  ClientId=parClientId  ConnectionId=parConnectionId  Topic='port0/ci/ev/parameter/mincurrentlimit'  QoS=0 - at most once  Retain=on  Extended=off  SampleTime=parSampleTime
      settings: SourceProductName=MQTT
  port0_ci_ev_parameter_resssoc : speedgoatlib_mqtt/Client/MQTT Client Publish  ClientId=parClientId  ConnectionId=parConnectionId  Topic='port0/ci/ev/parameter/resssoc'  QoS=0 - at most once  Retain=on  Extended=off  SampleTime=parSampleTime
      settings: SourceProductName=MQTT
  to physical value format : MATLAB Function  TreatAsAtomicUnit=on
  to physical value format1 : MATLAB Function  TreatAsAtomicUnit=on
  to physical value format2 : MATLAB Function  TreatAsAtomicUnit=on
  to physical value format3 : MATLAB Function  TreatAsAtomicUnit=on
  to physical value format4 : MATLAB Function  TreatAsAtomicUnit=on
  to physical value format5 : MATLAB Function  TreatAsAtomicUnit=on
  wires:
  Function Caller/1 -> port0_ci_ev_parameter_maxvoltagelimit/1
  String to ASCII5/1 -> port0_ci_ev_parameter_resssoc/1
  To String1/1 -> String to ASCII5/1
  To String2/1 -> String to ASCII7/1
  String to ASCII7/1 -> port0_ci_ev_parameter_fullsoc/1
  String to ASCII8/1 -> port0_ci_ev_parameter_bulksoc/1
  To String3/1 -> String to ASCII8/1
  To String8/1 -> String to ASCII16/1
  String to ASCII16/1 -> port0_ci_ev_parameter_departuretime/1
  maxvoltagelimit/1 -> to physical value format/1(input)
  maxcurrentlimit/1 -> to physical value format1/1(input)
  mincurrentlimit/1 -> to physical value format2/1(input)
  maxpowerlimit/1 -> to physical value format3/1(input)
  energycapacity/1 -> to physical value format4/1(input)
  energyrequest/1 -> to physical value format5/1(input)
  bulksoc/1 -> To String3/1
  to physical value format/1(multiplier) -> Function Caller/1
  to physical value format/2(value) -> Function Caller/2
  ressoc/1 -> To String1/1
  fullsoc/1 -> To String2/1
  departuretime/1 -> To String8/1
  to physical value format1/2(value) -> Function Caller1/2
  to physical value format1/1(multiplier) -> Function Caller1/1
  Function Caller1/1 -> port0_ci_ev_parameter_maxcurrentlimit/1
  Function Caller2/1 -> port0_ci_ev_parameter_mincurrentlimit/1
  to physical value format2/1(multiplier) -> Function Caller2/1
  to physical value format2/2(value) -> Function Caller2/2
  to physical value format3/2(value) -> Function Caller3/2
  to physical value format3/1(multiplier) -> Function Caller3/1
  Function Caller3/1 -> port0_ci_ev_parameter_maxpowerlimit/1
  Function Caller4/1 -> port0_ci_ev_parameter_energycapacity/1
  to physical value format4/1(multiplier) -> Function Caller4/1
  to physical value format4/2(value) -> Function Caller4/2
  to physical value format5/2(value) -> Function Caller5/2
  to physical value format5/1(multiplier) -> Function Caller5/1
  Function Caller5/1 -> port0_ci_ev_parameter_energyrequest/1

== system speedgoatlib_evse/Blocks by Charge State/EV Setup /string compare logic ==
  Input : Inport
  ASCII to String1 : ASCIIToString
  Add : Sum
  Data Type Conversion : DataTypeConversion  OutDataTypeStr=double  SaturateOnIntegerOverflow=off  RndMeth=Floor
  Data Type Conversion1 : DataTypeConversion  OutDataTypeStr=double  SaturateOnIntegerOverflow=off  RndMeth=Floor
  Gain : Gain  Gain=2
  String Compare : StringCompare
  String Compare1 : StringCompare
  String Constant : StringConstant  String="\"started\""
  String Constant1 : StringConstant  String="\"finished\""
  Out1 : Outport
  wires:
  ASCII to String1/1 -> String Compare1/1, String Compare/1
  String Constant1/1 -> String Compare1/2
  String Compare/1 -> Data Type Conversion/1
  String Constant/1 -> String Compare/2
  String Compare1/1 -> Data Type Conversion1/1
  Gain/1 -> Add/2
  Add/1 -> Out1/1
  Input/1 -> ASCII to String1/1
  Data Type Conversion/1 -> Add/1
  Data Type Conversion1/1 -> Gain/1

== system speedgoatlib_evse/Blocks by Charge State/EV Stop Read /Enabled Subsystem ==
  Enable : EnablePort
  ASCII to String : ASCIIToString
  ASCII to String1 : ASCIIToString
  Data Type Conversion1 : DataTypeConversion  OutDataTypeStr=boolean  SaturateOnIntegerOverflow=off  RndMeth=Floor
  String to Double1 : ScanString  Format="\"%lf\""
  String to Double2 : ScanString  Format="\"%lf\""
  port0_ci_evse_stop_evseprocessing : speedgoatlib_mqtt/Client/MQTT Client Subscribe  ClientId=parClientId  ConnectionId=parConnectionId  Topic='port0/ci/evse/stop/evseprocessing'  QoS=0 - at most once  InitValue=zeros(1,12,'uint8')  Extended=off  SampleTime=parSampleTime
      settings: SourceProductName=MQTT
  port0_ci_evse_stop_progress : speedgoatlib_mqtt/Client/MQTT Client Subscribe  ClientId=parClientId  ConnectionId=parConnectionId  Topic='port0/ci/evse/stop/progress'  QoS=0 - at most once  InitValue=zeros(1,12,'uint8')  Extended=off  SampleTime=parSampleTime
      settings: SourceProductName=MQTT
  EVSE Stop Progress : Outport
  EVSE Processing : Outport  Port=2
  wires:
  Data Type Conversion1/1 -> EVSE Stop Progress/1
  port0_ci_evse_stop_progress/1 -> ASCII to String1/1
  String to Double1/1 -> Data Type Conversion1/1
  ASCII to String1/1 -> String to Double1/1
  port0_ci_evse_stop_evseprocessing/1 -> ASCII to String/1
  String to Double2/1 -> EVSE Processing/1
  ASCII to String/1 -> String to Double2/1

== system speedgoatlib_evse/Blocks by Charge State/EV Stop Read /string compare logic ==
  Input : Inport
  ASCII to String1 : ASCIIToString
  Add : Sum
  Gain : Gain  Gain=2
  String Compare : StringCompare
  String Compare1 : StringCompare
  String Constant : StringConstant  String="\"started\""
  String Constant1 : StringConstant  String="\"finished\""
  Out1 : Outport
  wires:
  ASCII to String1/1 -> String Compare1/1, String Compare/1
  String Constant1/1 -> String Compare1/2
  String Compare/1 -> Add/1
  String Constant/1 -> String Compare/2
  String Compare1/1 -> Gain/1
  Gain/1 -> Add/2
  Add/1 -> Out1/1
  Input/1 -> ASCII to String1/1

== system speedgoatlib_evse/Blocks by Charge State/EV Stop Write /Enabled Subsystem ==
  stopProgress : Inport
  Enable : EnablePort
  Constant5 : Constant  Value=parEnStopProgress  OutDataTypeStr=boolean
  Data Type Conversion1 : DataTypeConversion  OutDataTypeStr=double  SaturateOnIntegerOverflow=off  RndMeth=Floor
  Ground5 : Ground
  String to ASCII2 : StringToASCII  OutputVectorSize=12
  To String2 : ToString
  port0_ci_ev_stop_progress : speedgoatlib_mqtt/Client/MQTT Client Publish  ClientId=parClientId  ConnectionId=parConnectionId  Topic='port0/ci/ev/stop/progress'  QoS=0 - at most once  Retain=on  Extended=on  SampleTime=parSampleTime
      settings: SourceProductName=MQTT
  wires:
  stopProgress/1 -> Data Type Conversion1/1
  Data Type Conversion1/1 -> To String2/1
  To String2/1 -> String to ASCII2/1
  String to ASCII2/1 -> port0_ci_ev_stop_progress/1
  Ground5/1 -> port0_ci_ev_stop_progress/3
  Constant5/1 -> port0_ci_ev_stop_progress/2

== system speedgoatlib_evse/Blocks by Charge State/EV Stop Write /string compare logic ==
  Input : Inport
  ASCII to String1 : ASCIIToString
  Add : Sum
  Gain : Gain  Gain=2
  String Compare : StringCompare
  String Compare1 : StringCompare
  String Constant : StringConstant  String="\"started\""
  String Constant1 : StringConstant  String="\"finished\""
  Out1 : Outport
  wires:
  Input/1 -> ASCII to String1/1
  Add/1 -> Out1/1
  Gain/1 -> Add/2
  String Compare1/1 -> Gain/1
  String Constant/1 -> String Compare/2
  String Compare/1 -> Add/1
  String Constant1/1 -> String Compare1/2
  ASCII to String1/1 -> String Compare/1, String Compare1/1

== system speedgoatlib_evse/Blocks by Charge State/EV Welding Read /Enabled Subsystem ==
  Enable : EnablePort
  ASCII to String1 : ASCIIToString
  ASCII to String2 : ASCIIToString
  ASCII to String3 : ASCIIToString
  Data Type Conversion3 : DataTypeConversion  OutDataTypeStr=boolean  SaturateOnIntegerOverflow=off  RndMeth=Floor
  Data Type Conversion4 : DataTypeConversion  OutDataTypeStr=boolean  SaturateOnIntegerOverflow=off  RndMeth=Floor
  Function Caller : FunctionCaller  FunctionPrototype=value = fromJsonPhysicalValue(uint8_vec)  InputArgumentSpecifications=zeros(1,48,'uint8')  OutputArgumentSpecifications=double(0)
  Simulink Function : Subsystem  TreatAsAtomicUnit=on
  String to Double : ScanString  Format="\"%lf\""
  String to Double1 : ScanString  Format="\"%lf\""
  String to Double2 : ScanString  Format="\"%lf\""
  port0_ci_evse_welding_isolationstatus : speedgoatlib_mqtt/Client/MQTT Client Subscribe  ClientId=parClientId  ConnectionId=parConnectionId  Topic='port0/ci/evse/welding/isolationstatus'  QoS=0 - at most once  InitValue=zeros(1,12,'uint8')  Extended=off  SampleTime=parSampleTime
      settings: SourceProductName=MQTT
  port0_ci_evse_welding_notification : speedgoatlib_mqtt/Client/MQTT Client Subscribe  ClientId=parClientId  ConnectionId=parConnectionId  Topic='port0/ci/evse/welding/notification'  QoS=0 - at most once  InitValue=zeros(1,16,'uint8')  Extended=off  SampleTime=parSampleTime
      settings: SourceProductName=MQTT
  port0_ci_evse_welding_presentvoltage : speedgoatlib_mqtt/Client/MQTT Client Subscribe  ClientId=parClientId  ConnectionId=parConnectionId  Topic='port0/ci/evse/welding/presentvoltage'  QoS=0 - at most once  InitValue=zeros(1,48,'uint8')  Extended=off  SampleTime=parSampleTime
      settings: SourceProductName=MQTT
  port0_ci_evse_welding_statuscode : speedgoatlib_mqtt/Client/MQTT Client Subscribe  ClientId=parClientId  ConnectionId=parConnectionId  Topic='port0/ci/evse/welding/statuscode'  QoS=0 - at most once  InitValue=zeros(1,12,'uint8')  Extended=off  SampleTime=parSampleTime
      settings: SourceProductName=MQTT
  EVSE Notification : Outport
  EVSE Isolation Status : Outport  Port=2
  EVSE Statuscode : Outport  Port=3
  EVSE Present Voltage : Outport  Port=4
  wires:
  port0_ci_evse_welding_notification/1 -> ASCII to String1/1
  String to Double1/1 -> EVSE Notification/1
  ASCII to String1/1 -> String to Double1/1
  String to Double2/1 -> Data Type Conversion4/1
  ASCII to String2/1 -> String to Double2/1
  Data Type Conversion4/1 -> EVSE Isolation Status/1
  port0_ci_evse_welding_isolationstatus/1 -> ASCII to String2/1
  port0_ci_evse_welding_statuscode/1 -> ASCII to String3/1
  ASCII to String3/1 -> String to Double/1
  String to Double/1 -> Data Type Conversion3/1
  Data Type Conversion3/1 -> EVSE Statuscode/1
  Function Caller/1 -> EVSE Present Voltage/1
  port0_ci_evse_welding_presentvoltage/1 -> Function Caller/1
